simulink model "foc_system"  (R2026a)
settings: Solver=VariableStepAuto  StopTime=.1  FixedStep=1/20e3  MaxStep=1/20e3
PreLoadFcn:
  | try, p = fileparts(which(bdroot)); addpath(fullfile(p,'..', 'scripts')); addpath(fullfile(p,'..', 'models')); addpath(p); catch, end; init;
InitFcn:
  | try, p = fileparts(which(bdroot)); addpath(fullfile(p,'..', 'scripts')); addpath(fullfile(p,'..', 'models')); addpath(p); catch, end; init;
settings Model: Creator=probst  LastModifiedBy=probst
settings DebuggingCC: ParameterPrecisionLossMsg=none

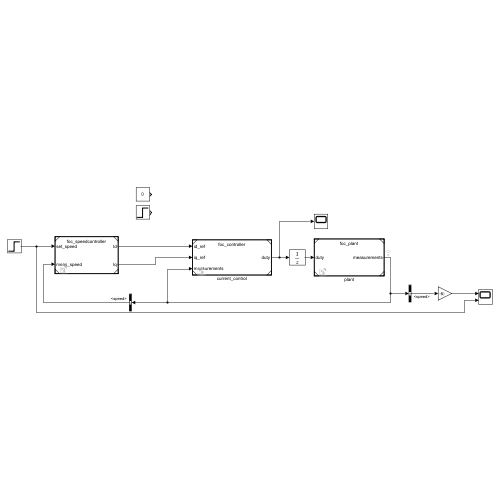
[thumbnail: Simulink's stored preview of the top-level diagram]
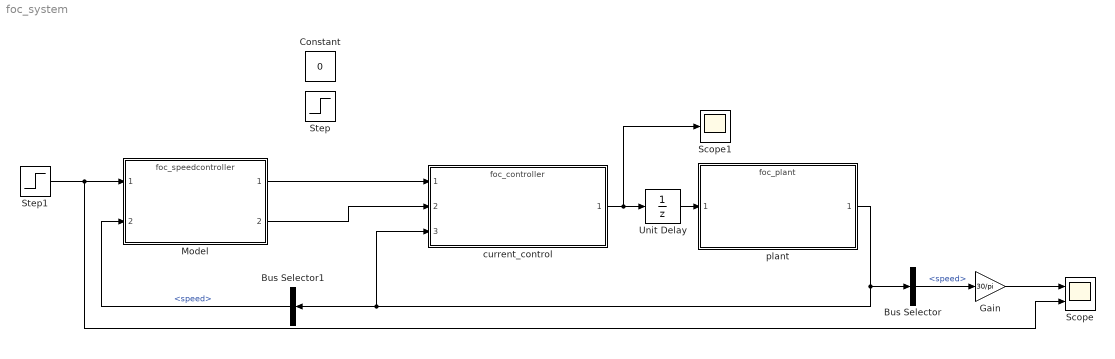
== system foc_system ==
  Bus Selector : BusSelector  OutputSignals=speed
  Bus Selector1 : BusSelector  OutputSignals=speed
  Constant : Constant  Value=0
  Gain : Gain  Gain=30/pi
  Model : ModelReference  ModelNameDialog=foc_speedcontroller.slx  SimulationMode=Normal  ModelReferenceVersion=1.5
  Scope : Scope  NumInputPorts=2
      settings: ActiveDisplayYMinimum=-75.098932663651425  ActiveDisplayYMaximum=675.890393972863
  Scope1 : Scope
      settings: ActiveDisplayYMinimum=-0.082279583221092523  ActiveDisplayYMaximum=1.0175814133106607
  Step : Step  Time=.1  FinalValue=50  SampleTime=0
  Step1 : Step  Time=.05  FinalValue=600  SampleTime=0
  Unit Delay : UnitDelay  SampleTime=-1
  current_control : ModelReference  ModelNameDialog=foc_controller.slx  SimulationMode=Normal  ModelReferenceVersion=1.67
  plant : ModelReference  ModelNameDialog=foc_plant.slx  SimulationMode=Normal  ModelReferenceVersion=1.39
  wires:
  plant/1 -> current_control/3, Bus Selector1/1, Bus Selector/1
  Bus Selector/1 -> Gain/1  "<speed>"
  current_control/1 -> Unit Delay/1, Scope1/1
  Bus Selector1/1 -> Model/2  "<speed>"
  Step1/1 -> Scope/2, Model/1
  Model/1 -> current_control/1
  Model/2 -> current_control/2
  Gain/1 -> Scope/1
  Unit Delay/1 -> plant/1
